simulink model "Scenario_3_PF"  (R2020b)
settings: Solver=ode1  StartTime=0.0  StopTime=10.0  RelTol=1e-3
InitFcn:
  | Scenario_3_parameters;
values from neighbouring files (symbols this model uses):
  c0 = c0_zeb    (= 6.57988e-09)    [Scenario_17_parameters_v2.m]    (also in Scenario_1_parameters_v2.m; Scenario_2_parameters_v2.m; Scenario_3_parameters_v2.m)
  c0_hawk = 6.37282e-09    [Scenario_17_parameters_v2.m]    (also in Scenario_1_parameters_v2.m; Scenario_2_parameters_v2.m; Scenario_3_parameters_v2.m)
  c1 = c1_zeb    (= 9.15905e-09)    [Scenario_17_parameters_v2.m]    (also in Scenario_1_parameters_v2.m; Scenario_2_parameters_v2.m; Scenario_3_parameters_v2.m)
  c1_hawk = 8.76156e-09    [Scenario_17_parameters_v2.m]    (also in Scenario_1_parameters_v2.m; Scenario_2_parameters_v2.m; Scenario_3_parameters_v2.m)
  fg = 50    [Scenario_17_parameters_v2.m]    (also in Scenario_1_parameters_v2.m; Scenario_2_parameters_v2.m; Scenario_3_parameters_v2.m)
  G10gen = 0.90    (= 0.9)    [Scenario_3_parameters_v2.m]
  G12gen = 0.85    [Scenario_3_parameters_v2.m]
  G1gen = 0.4692    [Scenario_17_parameters_v2.m]    (also in Scenario_1_parameters_v2.m = 0.1; Scenario_2_parameters_v2.m = 0.298581; Scenario_3_parameters_v2.m = 0.65)
  G2gen = 0.80    (= 0.8)    [Scenario_1_parameters_v2.m]    (also in Scenario_2_parameters_v2.m = 0.7; Scenario_3_parameters_v2.m = 0.4)
  G3gen = 0.85    [Scenario_1_parameters_v2.m]    (also in Scenario_2_parameters_v2.m = 0.9; Scenario_3_parameters_v2.m = 0.6)
  G4gen = 0.65    [Scenario_3_parameters_v2.m]
  G5gen = 0.75    [Scenario_17_parameters_v2.m]    (also in Scenario_1_parameters_v2.m = 0.8; Scenario_2_parameters_v2.m = 0.8; Scenario_3_parameters_v2.m = 0.705)
  G6gen = 0.90    (= 0.9)    [Scenario_17_parameters_v2.m]    (also in Scenario_1_parameters_v2.m; Scenario_2_parameters_v2.m = 0.81797; Scenario_3_parameters_v2.m = 0.45)
  G7gen = 0.20    (= 0.2)    [Scenario_17_parameters_v2.m]    (also in Scenario_1_parameters_v2.m = 0.5227; Scenario_2_parameters_v2.m = 0.5098; Scenario_3_parameters_v2.m = 0.4)
  G8gen = 0.58    [Scenario_17_parameters_v2.m]    (also in Scenario_3_parameters_v2.m = 0.65)
  G9gen = 0.8833    [Scenario_17_parameters_v2.m]    (also in Scenario_3_parameters_v2.m = 0.9)
  Ihvpk = Ihv*sqrt(2)    [Scenario_17_parameters_v2.m]    (also in Scenario_1_parameters_v2.m; Scenario_2_parameters_v2.m; Scenario_3_parameters_v2.m)
  l0 = l0_zeb    (= 0.00368)    [Scenario_17_parameters_v2.m]    (also in Scenario_1_parameters_v2.m; Scenario_2_parameters_v2.m; Scenario_3_parameters_v2.m)
  l0_hawk = 0.00373    [Scenario_17_parameters_v2.m]    (also in Scenario_1_parameters_v2.m; Scenario_2_parameters_v2.m; Scenario_3_parameters_v2.m)
  l1 = l1_zeb    (= 0.00128)    [Scenario_17_parameters_v2.m]    (also in Scenario_1_parameters_v2.m; Scenario_2_parameters_v2.m; Scenario_3_parameters_v2.m)
  L10dem = 0.04    [Scenario_3_parameters_v2.m]
  L12dem = 0.01    [Scenario_17_parameters_v2.m]    (also in Scenario_3_parameters_v2.m = 0.02)
  L13dem = 0.01    [Scenario_3_parameters_v2.m]
  l1_hawk = 0.00133    [Scenario_17_parameters_v2.m]    (also in Scenario_1_parameters_v2.m; Scenario_2_parameters_v2.m; Scenario_3_parameters_v2.m)
  L1dem = 0.25    [Scenario_17_parameters_v2.m]    (also in Scenario_3_parameters_v2.m = 0.1)
  L3dem = 0.30    (= 0.3)    [Scenario_17_parameters_v2.m]    (also in Scenario_1_parameters_v2.m = 0.1; Scenario_2_parameters_v2.m = 0.1; Scenario_3_parameters_v2.m = 0.2)
  L6dem = 0.15    [Scenario_1_parameters_v2.m]    (also in Scenario_2_parameters_v2.m; Scenario_3_parameters_v2.m = 0.1)
  L7dem = 0.10    (= 0.1)    [Scenario_1_parameters_v2.m]    (also in Scenario_2_parameters_v2.m; Scenario_3_parameters_v2.m = 0.2)
  L9dem = 0.15    [Scenario_17_parameters_v2.m]    (also in Scenario_3_parameters_v2.m = 0.1)
  Pr = Sr*PF    (= 1600500000)    [Scenario_17_parameters_v2.m]    (also in Scenario_1_parameters_v2.m = 1472500000; Scenario_2_parameters_v2.m = 1805000000; Scenario_3_parameters_v2.m = 12740000000)
  Qr = sqrt(Sr^2 - Pr^2)    [Scenario_17_parameters_v2.m]    (also in Scenario_1_parameters_v2.m; Scenario_2_parameters_v2.m; Scenario_3_parameters_v2.m)
  r0 = r0_zeb    (= 0.39362)    [Scenario_17_parameters_v2.m]    (also in Scenario_1_parameters_v2.m; Scenario_2_parameters_v2.m; Scenario_3_parameters_v2.m)
  r0_hawk = 0.44587    [Scenario_17_parameters_v2.m]    (also in Scenario_1_parameters_v2.m; Scenario_2_parameters_v2.m; Scenario_3_parameters_v2.m)
  r1 = r1_zeb    (= 0.06862)    [Scenario_17_parameters_v2.m]    (also in Scenario_1_parameters_v2.m; Scenario_2_parameters_v2.m; Scenario_3_parameters_v2.m)
  r1_hawk = 0.12087    [Scenario_17_parameters_v2.m]    (also in Scenario_1_parameters_v2.m; Scenario_2_parameters_v2.m; Scenario_3_parameters_v2.m)
  Rtpu = Xtpu/40    (= 0.0025)    [Scenario_17_parameters_v2.m]    (also in Scenario_1_parameters_v2.m = 0.00375; Scenario_2_parameters_v2.m = 0.00375; Scenario_3_parameters_v2.m)
  S10non = 500e6    (= 500000000)    [Scenario_3_parameters_v2.m]
  S12non = 250e6    (= 250000000)    [Scenario_3_parameters_v2.m]
  S1non = 700e6    (= 700000000)    [Scenario_17_parameters_v2.m]    (also in Scenario_1_parameters_v2.m = 400000000; Scenario_2_parameters_v2.m = 400000000; Scenario_3_parameters_v2.m = 1000000000)
  S2non = 300e6    (= 300000000)    [Scenario_1_parameters_v2.m]    (also in Scenario_2_parameters_v2.m; Scenario_3_parameters_v2.m = 3000000000)
  S3non = 200e6    (= 200000000)    [Scenario_1_parameters_v2.m]    (also in Scenario_2_parameters_v2.m; Scenario_3_parameters_v2.m = 1000000000)
  S4non = 2000e6    (= 2000000000)    [Scenario_3_parameters_v2.m]
  S5non = 400e6    (= 400000000)    [Scenario_17_parameters_v2.m]    (also in Scenario_1_parameters_v2.m = 500000000; Scenario_2_parameters_v2.m = 500000000; Scenario_3_parameters_v2.m = 2000000000)
  S6non = 150e6    (= 150000000)    [Scenario_17_parameters_v2.m]    (also in Scenario_1_parameters_v2.m = 400000000; Scenario_2_parameters_v2.m = 400000000; Scenario_3_parameters_v2.m = 3000000000)
  S7non = 1500e6    (= 1500000000)    [Scenario_17_parameters_v2.m]    (also in Scenario_1_parameters_v2.m = 200000000; Scenario_2_parameters_v2.m = 200000000; Scenario_3_parameters_v2.m = 4000000000)
  S8non = 600e6    (= 600000000)    [Scenario_17_parameters_v2.m]    (also in Scenario_3_parameters_v2.m = 2000000000)
  S9non = 200e6    (= 200000000)    [Scenario_17_parameters_v2.m]    (also in Scenario_3_parameters_v2.m = 1500000000)
  tonvsc = 0    [Scenario_17_parameters_v2.m]    (also in Scenario_1_parameters_v2.m; Scenario_2_parameters_v2.m; Scenario_3_parameters_v2.m = 0.0001)
  Ts = 50e-6    (= 5e-05)    [Scenario_17_parameters_v2.m]    (also in Scenario_1_parameters_v2.m = 0.0002; Scenario_2_parameters_v2.m = 2e-05; Scenario_3_parameters_v2.m = 0.0001)
  Vhv = 220e3    (= 220000)    [Scenario_17_parameters_v2.m]    (also in Scenario_1_parameters_v2.m; Scenario_2_parameters_v2.m; Scenario_3_parameters_v2.m)
  Vmv = 22e3    (= 22000)    [Scenario_17_parameters_v2.m]    (also in Scenario_1_parameters_v2.m; Scenario_2_parameters_v2.m; Scenario_3_parameters_v2.m)
  wc1 = wsw1/10    (= 848.230016469)    [Scenario_17_parameters_v2.m]    (also in Scenario_1_parameters_v2.m; Scenario_2_parameters_v2.m; Scenario_3_parameters_v2.m)
  wdc1 = wc1/10    (= 84.8230016469)    [Scenario_17_parameters_v2.m]    (also in Scenario_1_parameters_v2.m; Scenario_2_parameters_v2.m; Scenario_3_parameters_v2.m)
  wpq1 = wc1/10    (= 84.8230016469)    [Scenario_17_parameters_v2.m]    (also in Scenario_1_parameters_v2.m; Scenario_2_parameters_v2.m; Scenario_3_parameters_v2.m)
  wsw1 = ksw1*2*pi*fg    (= 8482.30016469)    [Scenario_17_parameters_v2.m]    (also in Scenario_1_parameters_v2.m; Scenario_2_parameters_v2.m; Scenario_3_parameters_v2.m)
  Xtpu = 0.10    (= 0.1)    [Scenario_17_parameters_v2.m]    (also in Scenario_1_parameters_v2.m = 0.15; Scenario_2_parameters_v2.m = 0.15; Scenario_3_parameters_v2.m)
undefined symbols (not defined in the file or in its folder): D11, Delta, Kf, r, theta0
libraries: powerlib x426, simulink_extras x305, powerlib_meascontrol x139, pid_lib x109, eeGeneralControl x72, simulink x60, eeTransforms x54, spsFirstOrderFilterLib x36, eePwmGeneratorTwoLevel x9
(part 19 of 36)

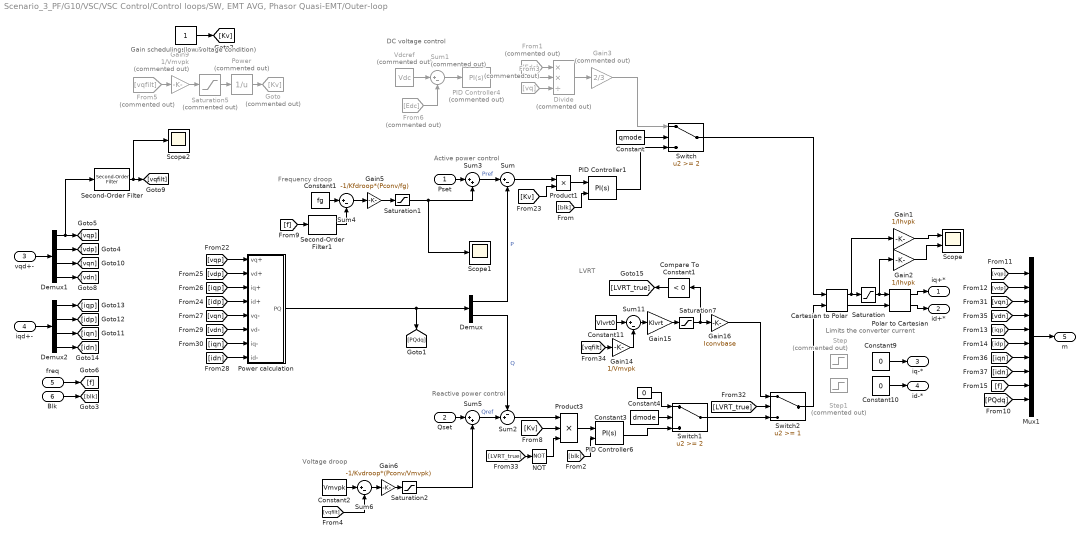
== system Scenario_3_PF/G10/VSC/VSC Control/Control loops/SW, EMT AVG, Phasor Quasi-EMT/Outer-loop ==
  note: Gain scheduling (low-voltage condition)
  note: DC voltage control
  note: Limits the converter current
  note: Frequency droop
  note: Voltage droop
  note: Reactive power control
  note: Active power control
  note: LVRT
  Pset : Inport
  Qset : Inport  Port=2
  vqd+- : Inport  Port=3
  iqd+- : Inport  Port=4
  freq : Inport  Port=5
  Blk : Inport  Port=6
  Cartesian to Polar : simulink_extras/Transformations/Cartesian to Polar
  Compare To Constant1 : simulink/Logic and Bit Operations/Compare To Constant  relop=<  const=0  OutDataTypeStr=boolean
  Constant : Constant  Value=qmode
  Constant1 : Constant  Value=fg
  Constant10 : Constant  Value=0
  Constant11 : Constant  Value=Vlvrt0
  Constant2 : Constant  Value=Vmvpk
  Constant3 : Constant  Value=dmode
  Constant4 : Constant  Value=0
  Constant8 : Constant
  Constant9 : Constant  Value=0
  Demux : Demux  Outputs=2
  Demux1 : Demux
  Demux2 : Demux
  Divide : Product  Commented=on  Inputs=**/
  From1 : From  Commented=on  GotoTag=Edc
  From3 : From  Commented=on  GotoTag=vq
  From5 : From  Commented=on  GotoTag=vqfilt
  From6 : From  Commented=on  GotoTag=Edc
  Gain1 : Gain  Gain=1/Ihvpk
  Gain14 : Gain  Gain=1/Vmvpk
  Gain15 : Gain  Gain=Klvrt
  Gain16 : Gain  Gain=Iconvbase
  Gain2 : Gain  Gain=1/Ihvpk
  Gain3 : Gain  Commented=on  Gain=2/3
  Gain5 : Gain  Gain=-1/Kfdroop*(Pconv/fg)
  Gain6 : Gain  Gain=-1/Kvdroop*(Pconv/Vmvpk)
  Gain9 : Gain  Commented=on  Gain=1/Vmvpk
  Goto : Goto  Commented=on  GotoTag=Kv
  Mux1 : Mux  Inputs=10
  NOT : Logic  Operator=NOT  IconShape=distinctive  AllPortsSameDT=off  OutDataTypeStr=boolean
  PID Controller1 : pid_lib/PID Controller  Controller=PI  Form=Ideal  TimeDomain=Continuous-time  UseExternalTs=off  SampleTime=-1  IntegratorMethod=Forward Euler  FilterMethod=Forward Euler  ControllerParametersSource=internal  P=kp_pq  I=1/ti_pq  D=0  UseFilter=on  N=100  TunerSelectOption=Transfer Function Based (PID Tuner App)  InitialConditionSource=internal  InitialConditionForIntegrator=0  InitialConditionForFilter=0  DifferentiatorICPrevScaledInput=0  ExternalReset=level  TrackingMode=off  Kt=1  LimitOutput=off  SatLimitsSource=internal  UpperSaturationLimit=inf  LowerSaturationLimit=-inf  LinearizeAsGain=on  AntiWindupMode=none  Kb=1  POutMin=[]  POutMax=[]  IOutMin=[]  IOutMax=[]  DOutMin=[]  DOutMax=[]  NOutMin=[]  NOutMax=[]  SumOutMin=[]  SumOutMax=[]  SaturationOutMin=[]  SaturationOutMax=[]  PParamMin=[]  PParamMax=[]  IParamMin=[]  IParamMax=[]  DParamMin=[]  DParamMax=[]  NParamMin=[]  NParamMax=[]  KbParamMin=[]  KbParamMax=[]  KtParamMin=[]  KtParamMax=[]  KbOutMin=[]  KbOutMax=[]  KtOutMin=[]  KtOutMax=[]  IntegratorOutMin=[]  IntegratorOutMax=[]  FilterOutMin=[]  FilterOutMax=[]  SumI1OutMin=[]  SumI1OutMax=[]  SumI2OutMin=[]  SumI2OutMax=[]  SumI3OutMin=[]  SumI3OutMax=[]  SumI4OutMin=[]  SumI4OutMax=[]  SumDOutMin=[]  SumDOutMax=[]  DifferentiatorOutMin=[]  DifferentiatorOutMax=[]  FilterDiffOutCoefMin=[]  FilterDiffOutCoefMax=[]  ReciprocalOutMin=[]  ReciprocalOutMax=[]  SumDenOutMin=[]  SumDenOutMax=[]  SumNumOutMin=[]  SumNumOutMax=[]  DivideOutMin=[]  DivideOutMax=[]  UdiffTsProdOutMin=[]  UdiffTsProdOutMax=[]  NTsProdOutMin=[]  NTsProdOutMax=[]  UintegralTsProdOutMin=[]  UintegralTsProdOutMax=[]  UngainTsProdOutMin=[]  UngainTsProdOutMax=[]  IntegratorContinuousStateAttributes=''  IntegratorStateMustResolveToSignalObject=off  IntegratorRTWStateStorageClass=Auto  FilterContinuousStateAttributes=''  FilterStateMustResolveToSignalObject=off  FilterRTWStateStorageClass=Auto  ParallelPVariant=Passthrough  IdealPVariant=InternalParameters  IVariant=InternalParameters  DVariant=Disabled  IntegratorVariant=Continuous  SatVariant=Disabled  AWVariant=Passthrough  PCopyVariant=Disabled  TRVariant=Disabled  FdbkBlocksVariant=Forward  IdealPFdbkVariant=Disabled  SatFdbkVariant=Disabled  DerivativeFilterVariant=Disabled  NVariant=Disabled  NCopyVariant=Disabled_SignalSpec  FilterICVariant=Disabled  IntegratorICVariant=InternalICs  ExternalResetVariant=ExternalReset  TRSumVariant=Passthrough  SumFdbkVariant=Disabled  SumVariant=Sum_PI  TsampFilterVariant=InternalTs  TsampNgainVariant=Passthrough  TsampIntegralVariant=Passthrough  ExternalSaturationOutDataTypeStr=Inherit: Same as second input
  PID Controller4 : pid_lib/PID Controller  Commented=on  Controller=PI  Form=Ideal  TimeDomain=Continuous-time  UseExternalTs=off  SampleTime=-1  IntegratorMethod=Forward Euler  FilterMethod=Forward Euler  ControllerParametersSource=internal  P=kp_dc  I=ki_dc/kp_dc  D=0  UseFilter=on  N=100  TunerSelectOption=Transfer Function Based (PID Tuner App)  InitialConditionSource=internal  InitialConditionForIntegrator=0  InitialConditionForFilter=0  DifferentiatorICPrevScaledInput=0  ExternalReset=none  TrackingMode=off  Kt=1  LimitOutput=off  SatLimitsSource=internal  UpperSaturationLimit=inf  LowerSaturationLimit=-inf  LinearizeAsGain=on  AntiWindupMode=none  Kb=1  POutMin=[]  POutMax=[]  IOutMin=[]  IOutMax=[]  DOutMin=[]  DOutMax=[]  NOutMin=[]  NOutMax=[]  SumOutMin=[]  SumOutMax=[]  SaturationOutMin=[]  SaturationOutMax=[]  PParamMin=[]  PParamMax=[]  IParamMin=[]  IParamMax=[]  DParamMin=[]  DParamMax=[]  NParamMin=[]  NParamMax=[]  KbParamMin=[]  KbParamMax=[]  KtParamMin=[]  KtParamMax=[]  KbOutMin=[]  KbOutMax=[]  KtOutMin=[]  KtOutMax=[]  IntegratorOutMin=[]  IntegratorOutMax=[]  FilterOutMin=[]  FilterOutMax=[]  SumI1OutMin=[]  SumI1OutMax=[]  SumI2OutMin=[]  SumI2OutMax=[]  SumI3OutMin=[]  SumI3OutMax=[]  SumI4OutMin=[]  SumI4OutMax=[]  SumDOutMin=[]  SumDOutMax=[]  DifferentiatorOutMin=[]  DifferentiatorOutMax=[]  FilterDiffOutCoefMin=[]  FilterDiffOutCoefMax=[]  ReciprocalOutMin=[]  ReciprocalOutMax=[]  SumDenOutMin=[]  SumDenOutMax=[]  SumNumOutMin=[]  SumNumOutMax=[]  DivideOutMin=[]  DivideOutMax=[]  UdiffTsProdOutMin=[]  UdiffTsProdOutMax=[]  NTsProdOutMin=[]  NTsProdOutMax=[]  UintegralTsProdOutMin=[]  UintegralTsProdOutMax=[]  UngainTsProdOutMin=[]  UngainTsProdOutMax=[]  IntegratorContinuousStateAttributes=''  IntegratorStateMustResolveToSignalObject=off  IntegratorRTWStateStorageClass=Auto  FilterContinuousStateAttributes=''  FilterStateMustResolveToSignalObject=off  FilterRTWStateStorageClass=Auto  ParallelPVariant=Passthrough  IdealPVariant=InternalParameters  IVariant=InternalParameters  DVariant=Disabled  IntegratorVariant=Continuous  SatVariant=Disabled  AWVariant=Passthrough  PCopyVariant=Disabled  TRVariant=Disabled  FdbkBlocksVariant=Forward  IdealPFdbkVariant=Disabled  SatFdbkVariant=Disabled  DerivativeFilterVariant=Disabled  NVariant=Disabled  NCopyVariant=Disabled_SignalSpec  FilterICVariant=Disabled  IntegratorICVariant=InternalICs  ExternalResetVariant=Disabled  TRSumVariant=Passthrough  SumFdbkVariant=Disabled  SumVariant=Sum_PI  TsampFilterVariant=InternalTs  TsampNgainVariant=Passthrough  TsampIntegralVariant=Passthrough  ExternalSaturationOutDataTypeStr=Inherit: Same as second input
  PID Controller6 : pid_lib/PID Controller  Controller=PI  Form=Ideal  TimeDomain=Continuous-time  UseExternalTs=off  SampleTime=-1  IntegratorMethod=Forward Euler  FilterMethod=Forward Euler  ControllerParametersSource=internal  P=kp_pq  I=1/ti_pq  D=0  UseFilter=on  N=100  TunerSelectOption=Transfer Function Based (PID Tuner App)  InitialConditionSource=internal  InitialConditionForIntegrator=0  InitialConditionForFilter=0  DifferentiatorICPrevScaledInput=0  ExternalReset=level  TrackingMode=off  Kt=1  LimitOutput=off  SatLimitsSource=internal  UpperSaturationLimit=inf  LowerSaturationLimit=-inf  LinearizeAsGain=on  AntiWindupMode=none  Kb=1  POutMin=[]  POutMax=[]  IOutMin=[]  IOutMax=[]  DOutMin=[]  DOutMax=[]  NOutMin=[]  NOutMax=[]  SumOutMin=[]  SumOutMax=[]  SaturationOutMin=[]  SaturationOutMax=[]  PParamMin=[]  PParamMax=[]  IParamMin=[]  IParamMax=[]  DParamMin=[]  DParamMax=[]  NParamMin=[]  NParamMax=[]  KbParamMin=[]  KbParamMax=[]  KtParamMin=[]  KtParamMax=[]  KbOutMin=[]  KbOutMax=[]  KtOutMin=[]  KtOutMax=[]  IntegratorOutMin=[]  IntegratorOutMax=[]  FilterOutMin=[]  FilterOutMax=[]  SumI1OutMin=[]  SumI1OutMax=[]  SumI2OutMin=[]  SumI2OutMax=[]  SumI3OutMin=[]  SumI3OutMax=[]  SumI4OutMin=[]  SumI4OutMax=[]  SumDOutMin=[]  SumDOutMax=[]  DifferentiatorOutMin=[]  DifferentiatorOutMax=[]  FilterDiffOutCoefMin=[]  FilterDiffOutCoefMax=[]  ReciprocalOutMin=[]  ReciprocalOutMax=[]  SumDenOutMin=[]  SumDenOutMax=[]  SumNumOutMin=[]  SumNumOutMax=[]  DivideOutMin=[]  DivideOutMax=[]  UdiffTsProdOutMin=[]  UdiffTsProdOutMax=[]  NTsProdOutMin=[]  NTsProdOutMax=[]  UintegralTsProdOutMin=[]  UintegralTsProdOutMax=[]  UngainTsProdOutMin=[]  UngainTsProdOutMax=[]  IntegratorContinuousStateAttributes=''  IntegratorStateMustResolveToSignalObject=off  IntegratorRTWStateStorageClass=Auto  FilterContinuousStateAttributes=''  FilterStateMustResolveToSignalObject=off  FilterRTWStateStorageClass=Auto  ParallelPVariant=Passthrough  IdealPVariant=InternalParameters  IVariant=InternalParameters  DVariant=Disabled  IntegratorVariant=Continuous  SatVariant=Disabled  AWVariant=Passthrough  PCopyVariant=Disabled  TRVariant=Disabled  FdbkBlocksVariant=Forward  IdealPFdbkVariant=Disabled  SatFdbkVariant=Disabled  DerivativeFilterVariant=Disabled  NVariant=Disabled  NCopyVariant=Disabled_SignalSpec  FilterICVariant=Disabled  IntegratorICVariant=InternalICs  ExternalResetVariant=ExternalReset  TRSumVariant=Passthrough  SumFdbkVariant=Disabled  SumVariant=Sum_PI  TsampFilterVariant=InternalTs  TsampNgainVariant=Passthrough  TsampIntegralVariant=Passthrough  ExternalSaturationOutDataTypeStr=Inherit: Same as second input
  Polar to Cartesian : simulink_extras/Transformations/Polar to Cartesian
      settings: SourceProductBaseCode=SL
  Power : Math  Commented=on  Operator=reciprocal  SaturateOnIntegerOverflow=on
  Power calculation : Subsystem
  Product1 : Product
  Product3 : Product  Inputs=3
  Saturation : Saturate  UpperLimit=Imax  LowerLimit=0
  Saturation1 : Saturate  UpperLimit=0.1*Pconv  LowerLimit=-0.1*Pconv
  Saturation2 : Saturate  UpperLimit=0.1*Pconv  LowerLimit=-0.1*Pconv
  Saturation5 : Saturate  Commented=on  UpperLimit=1.2  LowerLimit=0.2
  Saturation7 : Saturate  UpperLimit=0  LowerLimit=-Qmax_lvrt
  Scope : Scope  NumInputPorts=2
  Scope1 : Scope
  Scope2 : Scope
  Second-Order Filter : eeGeneralControl/Second-Order Filter  FilterType=Low-pass  fn=150  Zeta=0.9  Ts=-1  A0=0  Ph0=0  f0=0  b0=0
      settings: SourceProductBaseCode=PS
  Second-Order Filter1 : eeGeneralControl/Second-Order Filter  FilterType=Low-pass  fn=10  Zeta=0.9  Ts=-1  A0=50  Ph0=0  f0=0.001  b0=50
      settings: SourceProductBaseCode=PS
  Step : Step  Commented=on  Time=0.1  After=0.3*3711  SampleTime=0
  Step1 : Step  Commented=on  Time=0.2  After=0.2*3711  SampleTime=0
  Sum{,4,6,11} (4 alike) : Sum  Inputs=|+-
  Sum1 : Sum  Commented=on  Inputs=|+-
  Sum2 : Sum  Inputs=-+|
  Sum3 : Sum  Inputs=|++
  Sum5 : Sum  Inputs=|++
  Switch : Switch  Threshold=2
  Switch1 : Switch  Threshold=2
  Switch2 : Switch  Threshold=1
  Vdcref : Constant  Commented=on  Value=Vdc
  iq+* : Outport
  id+* : Outport  Port=2
  iq-* : Outport  Port=3
  id-* : Outport  Port=4
  m : Outport  Port=5
  wires:
  Constant4/1 -> Switch1/1
  Constant10/1 -> id-*/1
  Constant9/1 -> iq-*/1
  Second-Order Filter1/1 -> Sum4/2
  [f] -> Second-Order Filter1/1
  Saturation2/1 -> Sum5/2
  Qset/1 -> Sum5/1
  Cartesian to Polar/2 -> Polar to Cartesian/2
  Polar to Cartesian/1 -> iq+*/1
  Polar to Cartesian/2 -> id+*/1
  Cartesian to Polar/1 -> Gain1/1, Saturation/1
  Saturation/1 -> Gain2/1, Polar to Cartesian/1
  Demux/1 -> Sum/2  "P"
  Demux/2 -> Sum2/1  "Q"
  PID Controller1/1 -> Switch/3
  Constant/1 -> Switch/2
  Sum1/1 -> PID Controller4/1
  Divide/1 -> Gain3/1
  From1/1 -> Divide/1
  Vdcref/1 -> Sum1/1
  From6/1 -> Sum1/2
  PID Controller4/1 -> Divide/2
  Gain3/1 -> Switch/1
  Sum3/1 -> Sum/1  "Pref"
  Constant1/1 -> Sum4/1
  Gain5/1 -> Saturation1/1
  Sum4/1 -> Gain5/1
  Saturation1/1 -> Scope1/1, Sum3/2
  Sum5/1 -> Sum2/2  "Qref"
  Sum6/1 -> Gain6/1
  Gain6/1 -> Saturation2/1
  From3/1 -> Divide/3
  [vqfilt] -> Sum6/2
  Constant2/1 -> Sum6/1
  PID Controller6/1 -> Switch1/3
  Constant3/1 -> Switch1/2
  Sum/1 -> Product1/1
  [Kv] -> Product3/2
  Sum2/1 -> Product3/1
  Pset/1 -> Sum3/1
  Switch/1 -> Cartesian to Polar/1
  Blk/1 -> [blk]
  freq/1 -> [f]
  [vqp] -> Mux1/1
  Mux1/1 -> m/1
  Product3/1 -> PID Controller6/1
  Product1/1 -> PID Controller1/1
  From5/1 -> Gain9/1
  Gain9/1 -> Saturation5/1
  Saturation5/1 -> Power/1
  Power/1 -> Goto/1
  [Kv] -> Product1/2
  Second-Order Filter/1 -> Scope2/1, [vqfilt]
  Constant8/1 -> [Kv]
  vqd+-/1 -> Demux1/1
  iqd+-/1 -> Demux2/1
  Demux1/1 -> Second-Order Filter/1, [vqp]
  Demux1/2 -> [vdp]
  Demux1/3 -> [vqn]
  Demux1/4 -> [vdn]
  Demux2/1 -> [iqp]
  Demux2/2 -> [idp]
  Demux2/3 -> [iqn]
  Demux2/4 -> [idn]
  [vqp] -> Power calculation/1(vq+)
  [iqp] -> Power calculation/3(iq+)
  Power calculation/1(PQ) -> [PQdq], Demux/1
  [idp] -> Power calculation/4(id+)
  [vdp] -> Power calculation/2(vd+)
  [vqn] -> Power calculation/5(vq-)
  [vdn] -> Power calculation/6(vd-)
  [iqn] -> Power calculation/7(iq-)
  [idn] -> Power calculation/8(id-)
  [LVRT_true] -> NOT/1
  NOT/1 -> Product3/3
  [LVRT_true] -> Switch2/2
  Switch1/1 -> Switch2/3
  Switch2/1 -> Cartesian to Polar/2
  Compare To Constant1/1 -> [LVRT_true]
  Gain15/1 -> Saturation7/1
  Saturation7/1 -> Compare To Constant1/1, Gain16/1
  [vqfilt] -> Gain14/1
  Sum11/1 -> Gain15/1
  Gain14/1 -> Sum11/2
  Constant11/1 -> Sum11/1
  [vdp] -> Mux1/2
  [vqn] -> Mux1/3
  [vdn] -> Mux1/4
  [iqn] -> Mux1/7
  [idn] -> Mux1/8
  [f] -> Mux1/9
  [PQdq] -> Mux1/10
  [idp] -> Mux1/6
  [iqp] -> Mux1/5
  [blk] -> PID Controller1/2
  [blk] -> PID Controller6/2
  Gain16/1 -> Switch2/1
  Gain1/1 -> Scope/1
  Gain2/1 -> Scope/2

== system Scenario_3_PF/G10/VSC/VSC Control/Measurements/EMT/PLL aligned with positive-sequence ==
  note: PLL
      | aligned with vd+
  Vabc : Inport
  0-vd=-vd : Gain  Gain=-1
  Clock : Clock  Commented=on
  Constant : Constant  Commented=on  Value=2*pi*fg
  Constant1 : Constant  Commented=on  Value=2*pi
  Constant2 : Constant  Commented=on  Value=2*pi
  Filter : Constant  Commented=on  Value=-tfilt*fg*2*pi
  Gain : Gain  Gain=1/(2*pi)
  Integrator : Integrator
  Mod : Math  Commented=on  Operator=mod  SaturateOnIntegerOverflow=on
  Mod1 : Math  Commented=on  Operator=mod  SaturateOnIntegerOverflow=on
  Notch filter : Subsystem  Commented=through
  PID Controller : pid_lib/PID Controller  Commented=on  Controller=PI  Form=Ideal  TimeDomain=Continuous-time  UseExternalTs=off  SampleTime=-1  IntegratorMethod=Forward Euler  FilterMethod=Forward Euler  ControllerParametersSource=internal  P=kp_pll  I=1/tau_pll  D=0  UseFilter=on  N=100  TunerSelectOption=Transfer Function Based (PID Tuner App)  InitialConditionSource=internal  InitialConditionForIntegrator=2*pi*fg  InitialConditionForFilter=0  DifferentiatorICPrevScaledInput=0  ExternalReset=none  TrackingMode=off  Kt=1  LimitOutput=off  SatLimitsSource=internal  UpperSaturationLimit=1.1*2*pi*fg  LowerSaturationLimit=0.9*2*pi*fg  LinearizeAsGain=on  AntiWindupMode=clamping  Kb=1/kp_pll  POutMin=[]  POutMax=[]  IOutMin=[]  IOutMax=[]  DOutMin=[]  DOutMax=[]  NOutMin=[]  NOutMax=[]  SumOutMin=[]  SumOutMax=[]  SaturationOutMin=[]  SaturationOutMax=[]  PParamMin=[]  PParamMax=[]  IParamMin=[]  IParamMax=[]  DParamMin=[]  DParamMax=[]  NParamMin=[]  NParamMax=[]  KbParamMin=[]  KbParamMax=[]  KtParamMin=[]  KtParamMax=[]  KbOutMin=[]  KbOutMax=[]  KtOutMin=[]  KtOutMax=[]  IntegratorOutMin=[]  IntegratorOutMax=[]  FilterOutMin=[]  FilterOutMax=[]  SumI1OutMin=[]  SumI1OutMax=[]  SumI2OutMin=[]  SumI2OutMax=[]  SumI3OutMin=[]  SumI3OutMax=[]  SumI4OutMin=[]  SumI4OutMax=[]  SumDOutMin=[]  SumDOutMax=[]  DifferentiatorOutMin=[]  DifferentiatorOutMax=[]  FilterDiffOutCoefMin=[]  FilterDiffOutCoefMax=[]  ReciprocalOutMin=[]  ReciprocalOutMax=[]  SumDenOutMin=[]  SumDenOutMax=[]  SumNumOutMin=[]  SumNumOutMax=[]  DivideOutMin=[]  DivideOutMax=[]  UdiffTsProdOutMin=[]  UdiffTsProdOutMax=[]  NTsProdOutMin=[]  NTsProdOutMax=[]  UintegralTsProdOutMin=[]  UintegralTsProdOutMax=[]  UngainTsProdOutMin=[]  UngainTsProdOutMax=[]  IntegratorContinuousStateAttributes=''  IntegratorStateMustResolveToSignalObject=off  IntegratorRTWStateStorageClass=Auto  FilterContinuousStateAttributes=''  FilterStateMustResolveToSignalObject=off  FilterRTWStateStorageClass=Auto  ParallelPVariant=Passthrough  IdealPVariant=InternalParameters  IVariant=InternalParameters  DVariant=Disabled  IntegratorVariant=Continuous  SatVariant=Disabled  AWVariant=Passthrough  PCopyVariant=Disabled  TRVariant=Disabled  FdbkBlocksVariant=Forward  IdealPFdbkVariant=Disabled  SatFdbkVariant=Disabled  DerivativeFilterVariant=Disabled  NVariant=Disabled  NCopyVariant=Disabled_SignalSpec  FilterICVariant=Disabled  IntegratorICVariant=InternalICs  ExternalResetVariant=Disabled  TRSumVariant=Passthrough  SumFdbkVariant=Disabled  SumVariant=Sum_PI  TsampFilterVariant=InternalTs  TsampNgainVariant=Passthrough  TsampIntegralVariant=Passthrough  ExternalSaturationOutDataTypeStr=Inherit: Same as second input
  Park transform : Subsystem  Commented=on
  Phase-sequence separation : Subsystem
  Subsystem : Subsystem
      mask Display: disp('PI\n')
  Switch : Switch  Commented=on  Criteria=u2 > Threshold  Threshold=0.3
  Terminator : Terminator
  Terminator1 : Terminator
  Terminator2 : Terminator
  Transformer Y/D1 : Constant  Commented=on  Value=-pi/6
  theta : Outport
  f : Outport  Port=2
  wires:
  Integrator/1 -> theta/1, Phase-sequence separation/2(Theta)
  Constant2/1 -> Mod1/1
  Constant1/1 -> Mod/2
  Gain/1 -> f/1
  0-vd=-vd/1 -> Subsystem/1(in)
  Clock/1 -> Switch/2
  Constant/1 -> Switch/1
  Subsystem/1(w) -> Gain/1, Integrator/1
  Vabc/1 -> Phase-sequence separation/1(abc)
  Phase-sequence separation/1(q+) -> Terminator/1
  Phase-sequence separation/2(d+) -> 0-vd=-vd/1  "vd+"
  Phase-sequence separation/3(q-) -> Terminator1/1
  Phase-sequence separation/4(d-) -> Terminator2/1

== system Scenario_3_PF/G10/VSC/VSC Control/Measurements/EMT/Phase-sequence separation2 ==
  note: Phase-sequence separation based on
      | Delayed Signal Cancellation (DSC) method
  abc : Inport
  Theta : Inport  Port=2
  Complex to Real-Imag1 : ComplexToRealImag
  Complex to Real-Imag2 : ComplexToRealImag
  Complex to Real-Imag3 : ComplexToRealImag
  Constant : Constant  Value=negseq_en
  Demux3 : Demux  Outputs=3
  Exp2 : Math  OutputSignalType=complex  SaturateOnIntegerOverflow=on
  Exp3 : Math  OutputSignalType=complex  SaturateOnIntegerOverflow=on
  Gain1 : Gain  Gain=1/2
  Gain4 : Gain  Gain=-1i
  Gain5 : Gain  Gain=1i
  Gain6 : Gain  Gain=1/2
  Gain7 : Gain  Gain=1i
  NOT : Logic  Operator=NOT  IconShape=distinctive  AllPortsSameDT=off  OutDataTypeStr=boolean
  Product3 : Product
  Product4 : Product
  Real-Imag to Complex : RealImagToComplex
  Real-Imag to Complex1 : RealImagToComplex
  Sum1 : Sum  Inputs=|++
  Sum2 : Sum  Inputs=-+|
  Switch : Switch  Criteria=u2 ~= 0
  Terminator3 : Terminator
  Transport Delay2 : TransportDelay  DelayTime=1/4*(1/50)
  Transport Delay3 : TransportDelay  DelayTime=1/4*(1/50)
  abc to Alpha-Beta-Zero : powerlib_meascontrol/Transformations/abc to Alpha-Beta-Zero
  q+ : Outport
  d+ : Outport  Port=2
  q- : Outport  Port=3
  d- : Outport  Port=4
  wires:
  NOT/1 -> Switch/2
  Constant/1 -> NOT/1
  Switch/1 -> Product3/1
  Gain6/1 -> Switch/3
  Sum2/1 -> Gain1/1
  Transport Delay2/1 -> Real-Imag to Complex1/1
  Demux3/1 -> Real-Imag to Complex/1
  Complex to Real-Imag1/2 -> Transport Delay3/1
  Gain1/1 -> Product4/2
  Real-Imag to Complex/1 -> Complex to Real-Imag1/1, Sum2/2, Sum1/1, Switch/1
  Complex to Real-Imag3/1 -> d-/1
  Real-Imag to Complex1/1 -> Gain5/1
  Complex to Real-Imag1/1 -> Transport Delay2/1
  Transport Delay3/1 -> Real-Imag to Complex1/2
  Demux3/2 -> Real-Imag to Complex/2
  Product3/1 -> Complex to Real-Imag2/1
  Product4/1 -> Complex to Real-Imag3/1
  abc to Alpha-Beta-Zero/1 -> Demux3/1
  abc/1 -> abc to Alpha-Beta-Zero/1
  Exp3/1 -> Product4/1
  Complex to Real-Imag3/2 -> q-/1
  Complex to Real-Imag2/2 -> q+/1
  Demux3/3 -> Terminator3/1
  Sum1/1 -> Gain6/1
  Gain5/1 -> Sum2/1, Sum1/2
  Exp2/1 -> Product3/2
  Gain4/1 -> Exp2/1
  Theta/1 -> Gain4/1, Gain7/1
  Gain7/1 -> Exp3/1
  Complex to Real-Imag2/1 -> d+/1

== system Scenario_3_PF/G10/VSC/VSC Control/Measurements/EMT/Phase-sequence separation3 ==
  note: Phase-sequence separation based on
      | Delayed Signal Cancellation (DSC) method
  abc : Inport
  Theta : Inport  Port=2
  Complex to Real-Imag1 : ComplexToRealImag
  Complex to Real-Imag2 : ComplexToRealImag
  Complex to Real-Imag3 : ComplexToRealImag
  Constant : Constant  Value=negseq_en
  Demux3 : Demux  Outputs=3
  Exp2 : Math  OutputSignalType=complex  SaturateOnIntegerOverflow=on
  Exp3 : Math  OutputSignalType=complex  SaturateOnIntegerOverflow=on
  Gain1 : Gain  Gain=1/2
  Gain4 : Gain  Gain=-1i
  Gain5 : Gain  Gain=1i
  Gain6 : Gain  Gain=1/2
  Gain7 : Gain  Gain=1i
  NOT : Logic  Operator=NOT  IconShape=distinctive  AllPortsSameDT=off  OutDataTypeStr=boolean
  Product3 : Product
  Product4 : Product
  Real-Imag to Complex : RealImagToComplex
  Real-Imag to Complex1 : RealImagToComplex
  Sum1 : Sum  Inputs=|++
  Sum2 : Sum  Inputs=-+|
  Switch : Switch  Criteria=u2 ~= 0
  Terminator3 : Terminator
  Transport Delay2 : TransportDelay  DelayTime=1/4*(1/50)
  Transport Delay3 : TransportDelay  DelayTime=1/4*(1/50)
  abc to Alpha-Beta-Zero : powerlib_meascontrol/Transformations/abc to Alpha-Beta-Zero
  q+ : Outport
  d+ : Outport  Port=2
  q- : Outport  Port=3
  d- : Outport  Port=4
  wires:
  Complex to Real-Imag2/1 -> d+/1
  Gain7/1 -> Exp3/1
  Theta/1 -> Gain7/1, Gain4/1
  Gain4/1 -> Exp2/1
  Exp2/1 -> Product3/2
  Gain5/1 -> Sum1/2, Sum2/1
  Sum1/1 -> Gain6/1
  Demux3/3 -> Terminator3/1
  Complex to Real-Imag2/2 -> q+/1
  Complex to Real-Imag3/2 -> q-/1
  Exp3/1 -> Product4/1
  abc/1 -> abc to Alpha-Beta-Zero/1
  abc to Alpha-Beta-Zero/1 -> Demux3/1
  Product4/1 -> Complex to Real-Imag3/1
  Product3/1 -> Complex to Real-Imag2/1
  Demux3/2 -> Real-Imag to Complex/2
  Transport Delay3/1 -> Real-Imag to Complex1/2
  Complex to Real-Imag1/1 -> Transport Delay2/1
  Real-Imag to Complex1/1 -> Gain5/1
  Complex to Real-Imag3/1 -> d-/1
  Real-Imag to Complex/1 -> Switch/1, Sum1/1, Sum2/2, Complex to Real-Imag1/1
  Gain1/1 -> Product4/2
  Complex to Real-Imag1/2 -> Transport Delay3/1
  Demux3/1 -> Real-Imag to Complex/1
  Transport Delay2/1 -> Real-Imag to Complex1/1
  Sum2/1 -> Gain1/1
  Gain6/1 -> Switch/3
  Switch/1 -> Product3/1
  Constant/1 -> NOT/1
  NOT/1 -> Switch/2

== system Scenario_3_PF/G10/VSC/VSC Control/Measurements/Phasor/Frequency (Phasor)1 ==
  note: Calculates the frequency using the derivative of the voltage phase angle
  note: Zero the derivative in the first two time steps to avoid initialization peaks
  note: Avoid numerical peaks
      | Alternative to unwrap function
  Phase : Inport
  Constant : Constant  Value=fg
  Discrete Derivative : simulink/Discrete/Discrete Derivative  gainval=1.0  ICPrevScaledInput=0  OutMin=[]  OutMax=[]  OutDataType=fixdt(1, 16)  OutScaling=2^-10  DoSatur=off
  Gain1 : Gain  Gain=1/(2*pi)
  Product : Product
  Rate Limiter : RateLimiter  RisingSlewLimit=100  FallingSlewLimit=-100  SampleTimeMode=inherited
  Step : Step  Time=2*Ts  SampleTime=0
  Sum : Sum  Inputs=|++
  Freq : Outport
  wires:
  Phase/1 -> Discrete Derivative/1
  Gain1/1 -> Sum/1  "df"
  Constant/1 -> Sum/2
  Sum/1 -> Freq/1
  Step/1 -> Product/1
  Discrete Derivative/1 -> Product/2  "dw"
  Rate Limiter/1 -> Gain1/1
  Product/1 -> Rate Limiter/1

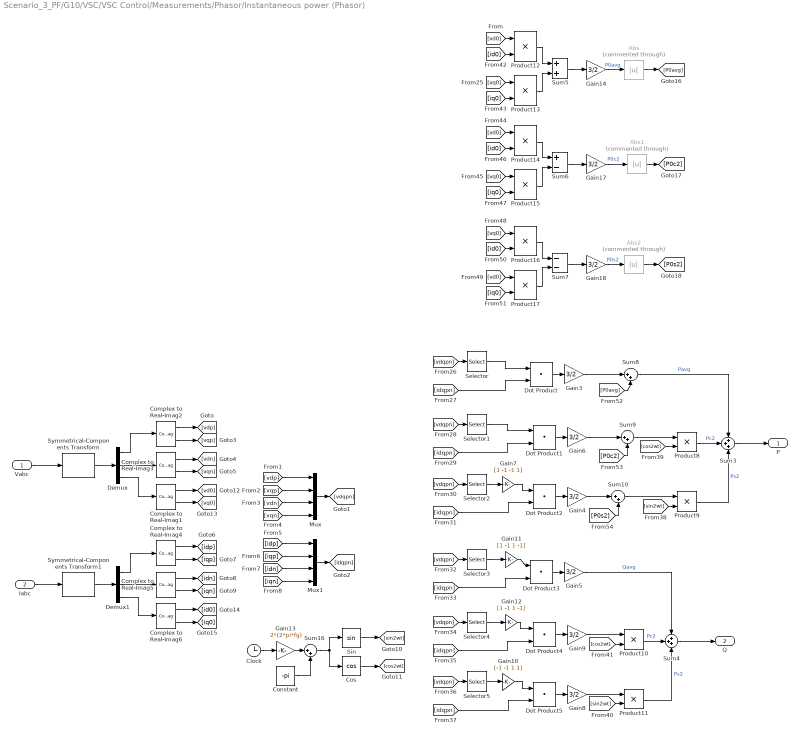
== system Scenario_3_PF/G10/VSC/VSC Control/Measurements/Phasor/Instantaneous power (Phasor) ==
  Vabc : Inport
  Iabc : Inport  Port=2
  Abs : Abs  Commented=through
  Abs1 : Abs  Commented=through
  Abs2 : Abs  Commented=through
  Clock : Clock
  Complex to Real-Imag{1..6} (6 alike) : ComplexToRealImag
  Constant : Constant  Value=-pi
  Cos : Trigonometry  Operator=cos
  Demux : Demux  Outputs=3
  Demux1 : Demux  Outputs=3
  Dot Product{,1..5} (6 alike) : DotProduct  InputSameDT=on  OutDataTypeStr=Inherit: Inherit via internal rule
  Gain10 : Gain  Gain=[-1 -1 1 1]
  Gain11 : Gain  Gain=[1 -1 1 -1]
  Gain12 : Gain  Gain=[1 -1 1 -1]
  Gain13 : Gain  Gain=2*(2*pi*fg)
  Gain{3..6,8..9,14,17..18} (9 alike) : Gain  Gain=3/2
  Gain7 : Gain  Gain=[1 -1 -1 1]
  Mux : Mux
  Mux1 : Mux
  Product{8..17} (10 alike) : Product
  Selector : Selector  InputPortWidth=4  IndexOptions=Index vector (dialog)  Indices=[1 2 3 4]  OutputSizes=1
  Selector1 : Selector  InputPortWidth=4  IndexOptions=Index vector (dialog)  Indices=[3 4 1 2]  OutputSizes=1
  Selector2 : Selector  InputPortWidth=4  IndexOptions=Index vector (dialog)  Indices=[4 3 2 1]  OutputSizes=1
  Selector3 : Selector  InputPortWidth=4  IndexOptions=Index vector (dialog)  Indices=[2 1 4 3]  OutputSizes=1
  Selector4 : Selector  InputPortWidth=4  IndexOptions=Index vector (dialog)  Indices=[4 3 2 1]  OutputSizes=1
  Selector5 : Selector  InputPortWidth=4  IndexOptions=Index vector (dialog)  Indices=[3 4 1 2]  OutputSizes=1
  Sin : Trigonometry
  Sum{8..10,16} (4 alike) : Sum  Inputs=|++
  Sum3 : Sum  Inputs=+++
  Sum4 : Sum  Inputs=+++
  Sum5 : Sum
  Sum6 : Sum  Inputs=+-
  Sum7 : Sum  Inputs=--
  Symmetrical-Components Transform : eeTransforms/Symmetrical-Components Transform  PowerInvariant=off
      settings: SourceProductBaseCode=PS
  Symmetrical-Components Transform1 : eeTransforms/Symmetrical-Components Transform  PowerInvariant=off
      settings: SourceProductBaseCode=PS
  P : Outport
  Q : Outport  Port=2
  wires:
  Abs2/1 -> [P0s2]
  Abs1/1 -> [P0c2]
  Complex to Real-Imag5/2 -> [iqn]
  Complex to Real-Imag3/2 -> [vqn]
  Complex to Real-Imag2/1 -> [vdp]
  Demux/1 -> Complex to Real-Imag2/1
  Complex to Real-Imag3/1 -> [vdn]
  Symmetrical-Components Transform1/1 -> Demux1/1
  Complex to Real-Imag2/2 -> [vqp]
  Symmetrical-Components Transform/1 -> Demux/1
  Complex to Real-Imag4/1 -> [idp]
  Complex to Real-Imag4/2 -> [iqp]
  Complex to Real-Imag5/1 -> [idn]
  Demux/2 -> Complex to Real-Imag3/1
  Demux1/2 -> Complex to Real-Imag5/1
  Demux1/1 -> Complex to Real-Imag4/1
  Iabc/1 -> Symmetrical-Components Transform1/1
  Vabc/1 -> Symmetrical-Components Transform/1
  Selector/1 -> Dot Product/1
  Dot Product/1 -> Gain3/1
  [vdp] -> Mux/1
  [vqp] -> Mux/2
  [vdn] -> Mux/3
  [vqn] -> Mux/4
  [idp] -> Mux1/1
  [iqp] -> Mux1/2
  [idn] -> Mux1/3
  [iqn] -> Mux1/4
  Mux/1 -> [vdqpn]
  Mux1/1 -> [idqpn]
  [vdqpn] -> Selector/1
  [idqpn] -> Dot Product/2
  [idqpn] -> Dot Product1/2
  Dot Product1/1 -> Gain6/1
  [vdqpn] -> Selector1/1
  Selector1/1 -> Dot Product1/1
  [idqpn] -> Dot Product2/2
  Dot Product2/1 -> Gain4/1
  [vdqpn] -> Selector2/1
  Selector2/1 -> Gain7/1
  Gain7/1 -> Dot Product2/1
  Sum3/1 -> P/1
  Gain10/1 -> Dot Product5/1
  [vdqpn] -> Selector3/1
  Gain5/1 -> Sum4/1  "Qavg"
  Dot Product5/1 -> Gain8/1
  Selector5/1 -> Gain10/1
  [vdqpn] -> Selector4/1
  [idqpn] -> Dot Product3/2
  Dot Product4/1 -> Gain9/1
  Dot Product3/1 -> Gain5/1
  [idqpn] -> Dot Product5/2
  Sum4/1 -> Q/1
  [idqpn] -> Dot Product4/2
  [vdqpn] -> Selector5/1
  Selector3/1 -> Gain11/1
  Gain11/1 -> Dot Product3/1
  Selector4/1 -> Gain12/1
  Gain12/1 -> Dot Product4/1
  Clock/1 -> Gain13/1
  Sin/1 -> [sin2wt]
  Cos/1 -> [cos2wt]
  Product8/1 -> Sum3/2  "Pc2"
  [cos2wt] -> Product8/2
  Product9/1 -> Sum3/3  "Ps2"
  [sin2wt] -> Product9/2
  [cos2wt] -> Product10/2
  [sin2wt] -> Product11/2
  Gain8/1 -> Product11/1
  Gain9/1 -> Product10/1
  Product10/1 -> Sum4/2  "Pc2"
  Product11/1 -> Sum4/3  "Ps2"
  Demux/3 -> Complex to Real-Imag1/1
  Complex to Real-Imag1/1 -> [vd0]
  Complex to Real-Imag1/2 -> [vq0]
  Complex to Real-Imag6/1 -> [id0]
  Complex to Real-Imag6/2 -> [iq0]
  Demux1/3 -> Complex to Real-Imag6/1
  [vd0] -> Product12/1
  [id0] -> Product12/2
  [iq0] -> Product13/2
  [vq0] -> Product13/1
  Product12/1 -> Sum5/1
  Product13/1 -> Sum5/2
  Sum5/1 -> Gain14/1
  Gain14/1 -> Abs/1  "P0avg"
  Sum6/1 -> Gain17/1
  [id0] -> Product14/2
  Product14/1 -> Sum6/1
  [iq0] -> Product15/2
  Gain17/1 -> Abs1/1  "P0c2"
  [vq0] -> Product15/1
  Product15/1 -> Sum6/2
  [vd0] -> Product14/1
  Sum7/1 -> Gain18/1
  [id0] -> Product16/2
  Product16/1 -> Sum7/1
  [iq0] -> Product17/2
  Gain18/1 -> Abs2/1  "P0s2"
  [vd0] -> Product17/1
  Product17/1 -> Sum7/2
  [vq0] -> Product16/1
  Sum8/1 -> Sum3/1  "Pavg"
  Gain3/1 -> Sum8/1
  [P0avg] -> Sum8/2
  Gain6/1 -> Sum9/1
  Sum9/1 -> Product8/1
  [P0c2] -> Sum9/2
  Gain4/1 -> Sum10/1
  Sum10/1 -> Product9/1
  [P0s2] -> Sum10/2
  Gain13/1 -> Sum16/1
  Constant/1 -> Sum16/2
  Sum16/1 -> Cos/1, Sin/1
  Abs/1 -> [P0avg]

== system Scenario_3_PF/G10/VSC/VSC Control/Measurements/Phasor/Subsystem ==
  note: ABC to symmetrical components
  abc : Inport
  Gain1 : Gain  Gain=[1 a a2]  SaturateOnIntegerOverflow=on  OutDataTypeStr=Inherit: Same as input  ParamDataTypeStr=Inherit: Same as input
  Gain2 : Gain  Gain=[1 a2 a]  SaturateOnIntegerOverflow=on  OutDataTypeStr=Inherit: Same as input  ParamDataTypeStr=Inherit: Same as input
  Gain5 : Gain  Gain=1/3  SaturateOnIntegerOverflow=on  OutDataTypeStr=Inherit: Same as input  ParamDataTypeStr=Inherit: Same as input
  Mux : Mux  Inputs=3
  Sum : Sum  Inputs=1  InputSameDT=on  SaturateOnIntegerOverflow=on  OutDataTypeStr=Inherit: Same as first input
  Sum1 : Sum  Inputs=1  InputSameDT=on  SaturateOnIntegerOverflow=on  OutDataTypeStr=Inherit: Same as first input
  Sum2 : Sum  Inputs=1  InputSameDT=on  SaturateOnIntegerOverflow=on  OutDataTypeStr=Inherit: Same as first input
  012 : Outport
  wires:
  Gain1/1 -> Sum/1
  abc/1 -> Gain2/1, Sum2/1, Gain1/1
  Gain2/1 -> Sum1/1
  Sum1/1 -> Mux/3
  Sum/1 -> Mux/2
  Sum2/1 -> Mux/1
  Mux/1 -> Gain5/1
  Gain5/1 -> 012/1

== system Scenario_3_PF/G10/VSC/VSC Control/Measurements/Phasor/Subsystem1 ==
  note: ABC to symmetrical components
  abc : Inport
  Gain1 : Gain  Gain=[1 a a2]  SaturateOnIntegerOverflow=on  OutDataTypeStr=Inherit: Same as input  ParamDataTypeStr=Inherit: Same as input
  Gain2 : Gain  Gain=[1 a2 a]  SaturateOnIntegerOverflow=on  OutDataTypeStr=Inherit: Same as input  ParamDataTypeStr=Inherit: Same as input
  Gain5 : Gain  Gain=1/3  SaturateOnIntegerOverflow=on  OutDataTypeStr=Inherit: Same as input  ParamDataTypeStr=Inherit: Same as input
  Mux : Mux  Inputs=3
  Sum : Sum  Inputs=1  InputSameDT=on  SaturateOnIntegerOverflow=on  OutDataTypeStr=Inherit: Same as first input
  Sum1 : Sum  Inputs=1  InputSameDT=on  SaturateOnIntegerOverflow=on  OutDataTypeStr=Inherit: Same as first input
  Sum2 : Sum  Inputs=1  InputSameDT=on  SaturateOnIntegerOverflow=on  OutDataTypeStr=Inherit: Same as first input
  012 : Outport
  wires:
  Gain1/1 -> Sum/1
  abc/1 -> Gain2/1, Sum2/1, Gain1/1
  Gain2/1 -> Sum1/1
  Sum1/1 -> Mux/3
  Sum/1 -> Mux/2
  Sum2/1 -> Mux/1
  Mux/1 -> Gain5/1
  Gain5/1 -> 012/1

== system Scenario_3_PF/G10/VSC/VSC Control/Measurements/Phasor/Subsystem3 ==
  abc : Inport
  Gain1 : Gain  Gain=[1 a a2]  SaturateOnIntegerOverflow=on  OutDataTypeStr=Inherit: Same as input  ParamDataTypeStr=Inherit: Same as input
  Gain3 : Gain  Gain=1/3  SaturateOnIntegerOverflow=on  OutDataTypeStr=Inherit: Same as input  ParamDataTypeStr=Inherit: Same as input
  Sum : Sum  Inputs=1  InputSameDT=on  SaturateOnIntegerOverflow=on  OutDataTypeStr=Inherit: Same as first input
  seq+ : Outport
  wires:
  Sum/1 -> Gain3/1
  abc/1 -> Gain1/1
  Gain1/1 -> Sum/1
  Gain3/1 -> seq+/1

== system Scenario_3_PF/G10/VSC/VSC Control/Modulation/EMT AVG/Corrects delay ==
  Clock : Clock
  Filter delay : Constant  Commented=on  Value=tfilt
  Gain : Gain  Gain=2*pi*fg
  Memory : Memory
  Sum : Sum  Inputs=|+-
  Sum1 : Sum  Inputs=|++
  Sum2 : Sum  Inputs=|++
  Transformer connection : Constant  Value=pi/6
  dphi : Outport
  wires:
  Clock/1 -> Memory/1, Sum/1
  Memory/1 -> Sum/2
  Sum1/1 -> Gain/1  "Td"
  Sum/1 -> Sum1/1  "Ts"
  Filter delay/1 -> Sum1/2  "Tf"
  Gain/1 -> Sum2/1
  Sum2/1 -> dphi/1
  Transformer connection/1 -> Sum2/2  "Tf"

== system Scenario_3_PF/G10/VSC/VSC Control/Modulation/EMT AVG/Corrects delay1 ==
  Clock : Clock
  Filter delay : Constant  Commented=on  Value=tfilt
  Gain : Gain  Gain=-2*pi*fg
  Gain1 : Gain
  Memory : Memory
  Sum : Sum  Inputs=|+-
  Sum1 : Sum  Inputs=|++
  Sum2 : Sum  Inputs=|++
  Transformer connection : Constant  Value=pi/6
  dphi : Outport
  wires:
  Clock/1 -> Memory/1, Sum/1
  Memory/1 -> Sum/2
  Sum1/1 -> Gain/1  "Td"
  Sum/1 -> Sum1/1  "Ts"
  Filter delay/1 -> Sum1/2  "Tf"
  Gain/1 -> Sum2/1
  Sum2/1 -> Gain1/1
  Transformer connection/1 -> Sum2/2  "Tf"
  Gain1/1 -> dphi/1

== system Scenario_3_PF/G10/VSC/VSC Control/Modulation/EMT Switching/Corrects delay ==
  Clock : Clock
  Filter delay : Constant  Commented=on  Value=tfilt
  Filter delay1 : Constant  Commented=on  Value=0.1*1/wsw1
  Gain : Gain  Gain=2*pi*fg
  Memory : Memory
  Sum : Sum  Inputs=|+-
  Sum1 : Sum  Inputs=+++
  Sum2 : Sum  Inputs=|++
  Transformer connection : Constant  Value=pi/6
  dphi : Outport
  wires:
  Sum2/1 -> dphi/1
  Transformer connection/1 -> Sum2/2  "Tf"
  Gain/1 -> Sum2/1
  Sum1/1 -> Gain/1  "Td"
  Memory/1 -> Sum/2
  Clock/1 -> Sum/1, Memory/1
  Sum/1 -> Sum1/2  "Ts"
  Filter delay/1 -> Sum1/3  "Tf"
  Filter delay1/1 -> Sum1/1  "Tf"

== system Scenario_3_PF/G10/VSC/VSC Control/Modulation/EMT Switching/Corrects delay1 ==
  Clock : Clock
  Filter delay : Constant  Commented=on  Value=tfilt
  Filter delay1 : Constant  Commented=on  Value=1/wsw1
  Gain : Gain  Gain=-2*pi*fg
  Memory : Memory
  Sum : Sum  Inputs=|+-
  Sum1 : Sum  Inputs=+++
  Sum2 : Sum  Inputs=|++
  Transformer connection : Constant  Value=pi/6
  dphi : Outport
  wires:
  Filter delay1/1 -> Sum1/1  "Tf"
  Filter delay/1 -> Sum1/3  "Tf"
  Sum/1 -> Sum1/2  "Ts"
  Clock/1 -> Memory/1, Sum/1
  Memory/1 -> Sum/2
  Sum1/1 -> Gain/1  "Td"
  Gain/1 -> Sum2/1
  Transformer connection/1 -> Sum2/2  "Tf"
  Sum2/1 -> dphi/1

== system Scenario_3_PF/G10/VSC/VSC Control/Modulation/Phasor I and Phasor PQ/Inverse Park Transform (Phasor) ==
  note: Transforming from real domain to complex domain
  note: In time domain, all variables are real.
      | In phasor domain, they are complex.
      | In phasor domain, what is seen as a variation in real domain is actually an angular displacement
      | As we know that the system is balanced, d and q have the same magnitude and are shifted 90 degrees
      | Thus, having the real parts and knowing that they are shifter 90 degrees, we can recover the complex part
  dq0 : Inport
  theta : Inport  Port=2
  Complex to Magnitude-Angle : ComplexToMagnitudeAngle  Commented=on
  Constant : Constant  Commented=on  Value=exp(-1i*2*pi/3)
  Constant1 : Constant  Commented=on  Value=exp(-1i*4*pi/3)
  Constant2 : Constant  Value=0
  Demux : Demux  Outputs=2
  Demux1 : Demux  Commented=on  Outputs=3
  Exp : Math  OutputSignalType=complex  SaturateOnIntegerOverflow=on
  Exp1 : Math  Commented=on  OutputSignalType=complex  SaturateOnIntegerOverflow=on
  First-Order Filter1 : spsFirstOrderFilterLib/First-Order Filter  Commented=on  FilterType=Lowpass  Tc=100e-6  Ts=0  Initialize=off  Vac_Init=[0, 0, 60]  Vdc_Init=0  PlotResponse=off  FreqRange="[0,  200,  1]"
  First-Order Filter2 : spsFirstOrderFilterLib/First-Order Filter  Commented=on  FilterType=Lowpass  Tc=100e-6  Ts=0  Initialize=off  Vac_Init=[0, 0, 60]  Vdc_Init=0  PlotResponse=off  FreqRange="[0,  200,  1]"
  Gain : Gain  Commented=on  Gain=exp(-1i*2*pi/3)
  Gain1 : Gain  Gain=1/2
  Gain2 : Gain  Gain=sqrt(3)
  Gain3 : Gain  Gain=1/2
  Gain4 : Gain  Gain=sqrt(3)
  Gain5 : Gain  Gain=1i
  Gain6 : Gain  Gain=-1
  Gain7 : Gain  Commented=on  Gain=1i
  Gain8 : Gain  Commented=on  Gain=exp(-1i*4*pi/3)
  Magnitude-Angle to Complex : MagnitudeAngleToComplex  Commented=on
  Mux : Mux  Commented=on  Inputs=3
  Mux2 : Mux  Inputs=3
  Product : Product
  Product1 : Product  Commented=on
  Real-Imag to Complex : RealImagToComplex
  Real-Imag to Complex1 : RealImagToComplex
  Sum : Sum  Inputs=|++
  Sum1 : Sum  Inputs=-|-
  Sum2 : Sum  Inputs=-|+
  Terminator : Terminator  Commented=on
  Terminator1 : Terminator  Commented=on
  abc : Outport  VectorParamsAs1DForOutWhenUnconnected=off
  wires:
  ? -> Demux1/1
  Demux1/3 -> Terminator1/1
  Magnitude-Angle to Complex/1 -> Gain/1, Mux/1, Gain8/1
  Gain/1 -> Mux/2
  Complex to Magnitude-Angle/1 -> First-Order Filter1/1
  Demux1/1 -> Complex to Magnitude-Angle/1
  Mux/1 -> ?
  Gain8/1 -> Mux/3
  Demux1/2 -> Terminator/1
  Complex to Magnitude-Angle/2 -> First-Order Filter2/1
  First-Order Filter2/1 -> Magnitude-Angle to Complex/2
  First-Order Filter1/1 -> Magnitude-Angle to Complex/1
  Sum/1 -> abc/1
  Constant2/1 -> [x0]
  Exp1/1 -> Product1/2
  Gain7/1 -> Exp1/1
  Gain6/1 -> Real-Imag to Complex1/2
  [xdr] -> Gain6/1
  [xqr] -> Real-Imag to Complex/2
  [xqr] -> Real-Imag to Complex1/1
  Real-Imag to Complex1/1 -> [xq]
  [xdr] -> Real-Imag to Complex/1
  Real-Imag to Complex/1 -> [xd]
  Gain3/1 -> Mux2/3
  Gain1/1 -> Mux2/2
  Sum2/1 -> Gain3/1
  [xd] -> Gain4/1
  [xq] -> Sum2/1
  Gain4/1 -> Sum2/2
  Gain2/1 -> Sum1/2
  [xd] -> Gain2/1
  [xq] -> Sum1/1
  Sum1/1 -> Gain1/1
  [xq] -> Mux2/1
  theta/1 -> Gain5/1
  Gain5/1 -> Exp/1
  Mux2/1 -> Product/1
  Exp/1 -> Product/2
  Product/1 -> Sum/1
  [x0] -> Sum/2
  Demux/2 -> [xqr]
  Demux/1 -> [xdr]
  dq0/1 -> Demux/1

== system Scenario_3_PF/G10/VSC/VSC Control/Modulation/Phasor I and Phasor PQ/RL time constant ==
  note: Adds an RL electrical time constant to the current source
  Id* : Inport
  Iq* : Inport  Port=2
  Cartesian to Polar : simulink_extras/Transformations/Cartesian to Polar
  Corrects delay : Subsystem  Commented=on
  Polar to Cartesian : simulink_extras/Transformations/Polar to Cartesian
      settings: SourceProductBaseCode=SL
  Saturation : Saturate  UpperLimit=Imax  LowerLimit=0
  Sum4 : Sum  Inputs=|++
  Transfer Fcn (with initial outputs) : simulink_extras/Additional Linear/Transfer Fcn (with initial outputs)  Commented=through  N=[1]  D=[L R]  Y0=0  U0=0
  Transfer Fcn (with initial outputs)1 : simulink_extras/Additional Linear/Transfer Fcn (with initial outputs)  Commented=through  N=[1]  D=[L R]  Y0=0  U0=0
  id : Outport  VectorParamsAs1DForOutWhenUnconnected=off
  iq : Outport  Port=2  VectorParamsAs1DForOutWhenUnconnected=off
  wires:
  Corrects delay/1(dphi) -> Sum4/2
  Sum4/1 -> Polar to Cartesian/2
  Cartesian to Polar/2 -> Sum4/1
  Id*/1 -> Transfer Fcn (with initial outputs)/1
  Iq*/1 -> Transfer Fcn (with initial outputs)1/1
  Polar to Cartesian/1 -> id/1
  Polar to Cartesian/2 -> iq/1
  Transfer Fcn (with initial outputs)/1 -> Cartesian to Polar/1
  Transfer Fcn (with initial outputs)1/1 -> Cartesian to Polar/2
  Cartesian to Polar/1 -> Saturation/1
  Saturation/1 -> Polar to Cartesian/1

== system Scenario_3_PF/G10/VSC/VSC Control/Modulation/Phasor I and Phasor PQ/Subsystem ==
  note: Symmetrical components to ABC
  012 : Inport
  Gain1 : Gain  Gain=[1 a a2]  SaturateOnIntegerOverflow=on  OutDataTypeStr=Inherit: Same as input  ParamDataTypeStr=Inherit: Same as input
  Gain2 : Gain  Gain=[1 a2 a]  SaturateOnIntegerOverflow=on  OutDataTypeStr=Inherit: Same as input  ParamDataTypeStr=Inherit: Same as input
  Mux : Mux  Inputs=3
  Sum : Sum  Inputs=1  InputSameDT=on  SaturateOnIntegerOverflow=on  OutDataTypeStr=Inherit: Same as first input
  Sum1 : Sum  Inputs=1  InputSameDT=on  SaturateOnIntegerOverflow=on  OutDataTypeStr=Inherit: Same as first input
  Sum2 : Sum  Inputs=1  InputSameDT=on  SaturateOnIntegerOverflow=on  OutDataTypeStr=Inherit: Same as first input
  abc : Outport
  wires:
  Mux/1 -> abc/1
  Sum2/1 -> Mux/1
  Sum/1 -> Mux/2
  Sum1/1 -> Mux/3
  Gain1/1 -> Sum1/1
  012/1 -> Gain2/1, Sum2/1, Gain1/1
  Gain2/1 -> Sum/1

== system Scenario_3_PF/G10/VSC/VSC Control/Modulation/Phasor Quasi-EMT/Corrects delay ==
  Clock : Clock
  Gain : Gain  Gain=(2*pi*fg)
  Memory : Memory
  Sum : Sum  Inputs=|+-
  Sum2 : Sum  Inputs=|++
  Transformer connection : Constant  Commented=on  Value=pi/6
  dphi : Outport
  wires:
  Clock/1 -> Memory/1, Sum/1
  Memory/1 -> Sum/2
  Sum/1 -> Gain/1  "Ts"
  Transformer connection/1 -> Sum2/2  "Tf"
  Gain/1 -> Sum2/1
  Sum2/1 -> dphi/1

== system Scenario_3_PF/G10/VSC/VSC Control/Modulation/Phasor Quasi-EMT/Corrects delay2 ==
  Clock : Clock
  Gain : Gain  Gain=(2*pi*fg)
  Memory : Memory
  Sum : Sum  Inputs=|+-
  Sum2 : Sum  Inputs=|++
  Transformer connection : Constant  Commented=on  Value=pi/6
  dphi : Outport
  wires:
  Clock/1 -> Memory/1, Sum/1
  Memory/1 -> Sum/2
  Sum/1 -> Gain/1  "Ts"
  Transformer connection/1 -> Sum2/2  "Tf"
  Gain/1 -> Sum2/1
  Sum2/1 -> dphi/1
